simulink model "PMSM_5_foc_smo5k_2019b"  (R2016a)
settings: Solver=ode45  StartTime=0.0  StopTime=0.8  FixedStep=1e-6  RelTol=1e-2
undefined symbols (not defined in the file or in its folder): Ls, Rs, udc
libraries: powerlib x7, simulink x4, powerlib_meascontrol x4
settings Model: Creator=Administrator  LastModifiedBy=Administrator

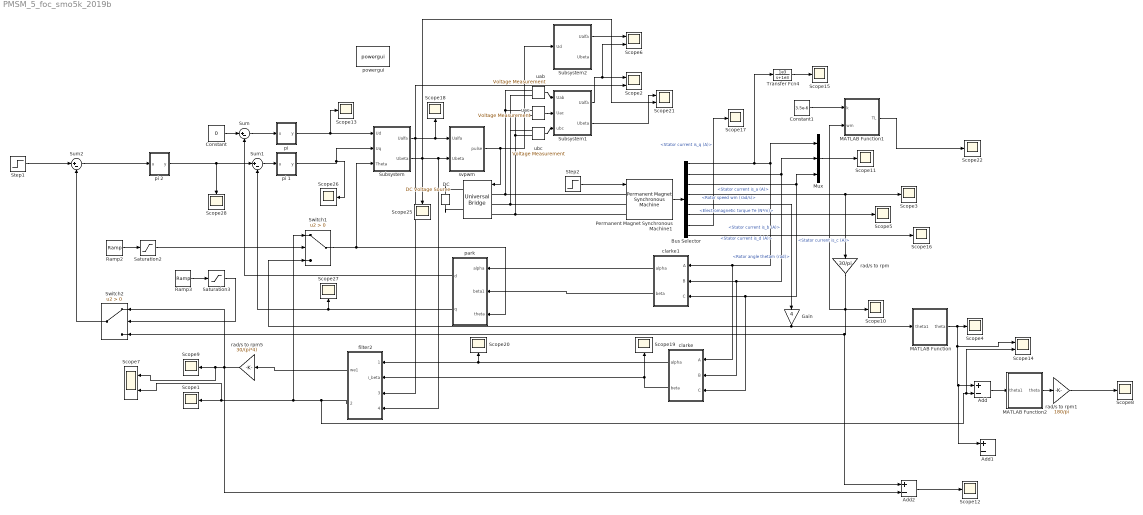
== system PMSM_5_foc_smo5k_2019b ==
  "   " : powerlib/Power Electronics/Universal Bridge  Arms=3  SnubberResistance=1e5  SnubberCapacitance=inf  Device=IGBT / Diodes  Ron=1e-3  Lon=0  ForwardVoltages="[  0  0  ]"  ForwardVoltage=0  GTOparameters=[ 10e-6 , 20e-6 ]  IGBTparameters=[ 1e-6 , 2e-6 ]  Measurements=All voltages and currents  Measurements_2=None  converterType=Rectifier
  " rad/s to rpm" : Gain  Gain=30/pi
  " rad/s to rpm1" : Gain  Gain=180/pi
  " rad/s to rpm5" : Gain  Gain=30/(pi*4)
  Add : Sum  Inputs=+-
  Add1 : Sum  Inputs=+-
  Add2 : Sum  Inputs=+-
  Bus Selector : BusSelector  OutputSignals=Stator current is_a (A),Stator current is_b (A),Stator current is_c (A),Rotor speed wm (rad/s),Rotor angle thetam (rad),Electromagnetic torque Te (N*m),Stator current is_q (A),Stator current is_d (A)
  Constant : Constant  Value=0
  Constant1 : Constant  Value=3.5e-6
  "DC " : powerlib/Electrical Sources/DC Voltage Source  Amplitude=280  Measurements=None
  Gain : Gain  Gain=4
  MATLAB Function : MATLAB Function  TreatAsAtomicUnit=on
  MATLAB Function1 : MATLAB Function  TreatAsAtomicUnit=on
  MATLAB Function2 : MATLAB Function  TreatAsAtomicUnit=on
  Mux : Mux  Inputs=3
  Permanent Magnet Synchronous Machine1 : powerlib/Machines/Permanent Magnet Synchronous Machine  NbPhases=3  FluxDistribution=Sinusoidal  RotorType=Salient-pole  MechanicalLoad=Torque Tm  PresetModel=No  ShowDetailedParameters=on  MeasurementBus=off  Resistance=0.1  Inductance=8.5e-3  dqInductances=[0.8e-3,0.8e-3]  La=1.6e-3  MachineConstant=Flux linkage established by magnets (V.s)  Flux=0.11  VoltageCst=79.8072  TorqueCst=0.66  Flat=120  Mechanical=[0.00223 0 4 0]  PolePairs=4  InitialConditions=[0,0, 0,0]  InitialConditions5ph=[0 0 0 0 0 0]  TsPowergui=0  TsBlock=-1  RefAngle=Aligned with phase A axis (original Park)
  Ramp2 : simulink/Sources/Ramp  slope=1  start=0  X0=-2
  Ramp3 : simulink/Sources/Ramp  slope=1  start=0  X0=-2
  Saturation2 : Saturate  UpperLimit=1  LowerLimit=0
  Saturation3 : Saturate  UpperLimit=1  LowerLimit=0
  Scope{1,3..5,8..13,15..20,22,25..28} (21 alike) : Scope
  Scope{2,6..7,14,21} (5 alike) : Scope  NumInputPorts=2
  Step1 : Step  Time=0.5  Before=400  After=400  SampleTime=0
  Step2 : Step  Time=0.3  Before=10  After=10  SampleTime=0
  Subsystem : Subsystem
  Subsystem1 : Subsystem
  Subsystem2 : Subsystem  InitFcn=udc=283
  Sum : Sum  Inputs=|+-
  Sum1 : Sum  Inputs=|+-
  Sum2 : Sum  Inputs=|+-
  Switch1 : Switch  Criteria=u2 > Threshold
  Switch2 : Switch  Criteria=u2 > Threshold
  Transfer Fcn4 : TransferFcn  Numerator=[1e3]  Denominator=[1 1e3]
  clarke : Subsystem
  clarke1 : Subsystem
  filter2 : Subsystem  InitFcn=|
      | Ls=0.8e-3
      | Rs=0.1
  park : Subsystem
  "pi " : Subsystem  mask{P=0.72, I=90, UpperSaturationLimit=280, LowerSaturationLimit=-280, SampleTime=-1}
  pi 1 : Subsystem  mask{P=0.72, I=90, UpperSaturationLimit=280, LowerSaturationLimit=-280, SampleTime=-1}
  pi 2 : Subsystem  mask{P=0.1061, I=10.6148, UpperSaturationLimit=30, LowerSaturationLimit=-30, SampleTime=-1}
  powergui : powerlib/powergui  Priority=1  SimulationMode=Continuous  SolverType=Backward Euler  SampleTime=1e-6  frequency=60  SPID=off  DisableSnubberDevices=off  DisableRonSwitches=off  DisableVfSwitches=off  SwTol=0  DisplayEquations=off  Interpol=off  ExternalGateDelay=off  methode=off  Ts=0  FunctionMessages=off  echomessages=off  HookPort=off  EnableUseOfTLC=off  x0status=blocks  frequencyindice=0  Pbase=100e6  ErrMax=1e-4  Iterations=50  UnitsV=kV  UnitsW=MW  buscounter=0  RestoreLinks=warning  ResistiveCurrentMeasurement=off  Frange=[0:2:500]  Ylog=off  Xlog=on  ShowGrid=off  save=off  variable=ZData  structure=smo5k_ia  ZoomFFT=off  StartTime=0.5  cycles=1  DisplayStyle=1  fundamental=200/3  FreqAxis=on  MaxFrequency=6000  frequencyindicesteady=1  RmsSteady=1  display=off
  svpwm : Subsystem  mask{T=1/2000, Udc=280, T_deadtime=0}
      mask prompts: T "T(s)"; Udc "Udc(V)"; T_deadtime "T_deadtime(us)"
  uab : powerlib/Measurements/Voltage Measurement  PhasorSimulation=off  OutputType=Complex  PSBequivalent=0
  uac : powerlib/Measurements/Voltage Measurement  PhasorSimulation=off  OutputType=Complex  PSBequivalent=0
  ubc : powerlib/Measurements/Voltage Measurement  PhasorSimulation=off  OutputType=Complex  PSBequivalent=0
  wires:
  svpwm/1(pulse) -> "   "/1, Subsystem2/1(Ud)
  Bus Selector/1 -> clarke/1(A), clarke1/1(A), Mux/1, Transfer Fcn4/1  "<Stator current is_a (A)>"
  Bus Selector/2 -> clarke/2(B), clarke1/2(B), Mux/2  "<Stator current is_b (A)>"
  Bus Selector/3 -> clarke/3(C), clarke1/3(C), Mux/3  "<Stator current is_c (A)>"
  Bus Selector/4 -> " rad/s to rpm"/1, Scope3/1  "<Rotor speed wm (rad/s)>"
  Bus Selector/5 -> Gain/1  "<Rotor angle thetam (rad)>"
  Bus Selector/6 -> Scope5/1  "<Electromagnetic torque Te (N*m)>"
  clarke/2(beta) -> Scope19/1, filter2/2(i_beta)
  Sum/1 -> "pi "/1(u)
  "pi "/1(y) -> Scope13/1, Subsystem/1(Ud)
  park/1(d) -> Sum/2
  Sum1/1 -> pi 1/1(u)
  Mux/1 -> Scope11/1
  Permanent Magnet Synchronous Machine1/1 -> Bus Selector/1
  Bus Selector/7 -> Scope17/1  "<Stator current is_q (A)>"
  Bus Selector/8 -> Scope16/1  "<Stator current is_d (A)>"
  Constant/1 -> Sum/1
  park/2(q) -> Sum1/2, Scope27/1
  pi 1/1(y) -> Scope26/1, Subsystem/2(Uq)
  pi 2/1(y) -> Sum1/1, Scope28/1
  filter2/1(we1) -> " rad/s to rpm5"/1
  Gain/1 -> MATLAB Function/1(theta1), Switch1/3
  " rad/s to rpm5"/1 -> Add2/2, Switch2/1, Scope7/1, Scope9/1
  filter2/2(theta*2) -> Scope14/2, Add/2, Switch1/1, Scope7/2, Scope1/1
  " rad/s to rpm"/1 -> MATLAB Function1/2(wm), Add2/1, Switch2/3, Scope10/1
  Step1/1 -> Sum2/1
  Switch2/1 -> Sum2/2
  Switch1/1 -> park/3(theta), Subsystem/3(Theta)
  Ramp2/1 -> Saturation2/1
  Saturation2/1 -> Switch1/2
  Ramp3/1 -> Saturation3/1
  Saturation3/1 -> Switch2/2
  clarke/1(alpha) -> Scope20/1, filter2/1(i_alpha)
  Transfer Fcn4/1 -> Scope15/1
  clarke1/1(alpha) -> park/1(alpha)
  clarke1/2(beta) -> park/2(beta1)
  uac/1 -> Subsystem1/2(Uac)
  uab/1 -> Subsystem1/1(Uab)
  ubc/1 -> Subsystem1/3(ubc)
  Subsystem1/1(Ualfa) -> Scope6/2, Scope2/1
  Subsystem1/2(Ubeta) -> Scope21/1
  Sum2/1 -> pi 2/1(u)
  Subsystem/1(Ualfa) -> svpwm/1(Ualfa), Scope18/1, filter2/3(u_alpha), Scope2/2
  Subsystem/2(Ubeta) -> Scope21/2, filter2/4(u_beta), svpwm/2(Ubeta), Scope25/1
  Step2/1 -> Permanent Magnet Synchronous Machine1/1
  Constant1/1 -> MATLAB Function1/1(k)
  MATLAB Function1/1(TL) -> Scope22/1
  Subsystem2/1(Ualfa) -> Scope6/1
  Add/1 -> MATLAB Function2/1(theta1)
  MATLAB Function/1(theta) -> Scope14/1, Add1/1, Add/1, Scope4/1
  Add2/1 -> Scope12/1
  MATLAB Function2/1(theta) -> " rad/s to rpm1"/1
  " rad/s to rpm1"/1 -> Scope8/1
  connections:
  "DC "/RConn1 -- "   "/RConn1
  Permanent Magnet Synchronous Machine1/LConn1 -- uab/LConn1 -- uac/LConn1 -- "   "/LConn1
  "DC "/LConn1 -- "   "/RConn2
  Permanent Magnet Synchronous Machine1/LConn3 -- ubc/LConn2 -- uac/LConn2 -- "   "/LConn3
  Permanent Magnet Synchronous Machine1/LConn2 -- ubc/LConn1 -- uab/LConn2 -- "   "/LConn2

== system PMSM_5_foc_smo5k_2019b/Subsystem ==
  Ud : Inport
  Uq : Inport  Port=2
  Theta : Inport  Port=3
  Fcn : Fcn  Expr=u(1)*cos(u(3))-u(2)*sin(u(3))
  Fcn1 : Fcn  Expr=u(1)*sin(u(3))+u(2)*cos(u(3))
  Mux : Mux  Inputs=3
  Mux1 : Mux  Inputs=3
  Ualfa : Outport
  Ubeta : Outport  Port=2
  wires:
  Ud/1 -> Mux1/1, Mux/1
  Uq/1 -> Mux1/2, Mux/2
  Theta/1 -> Mux1/3, Mux/3
  Mux/1 -> Fcn/1
  Mux1/1 -> Fcn1/1
  Fcn/1 -> Ualfa/1
  Fcn1/1 -> Ubeta/1

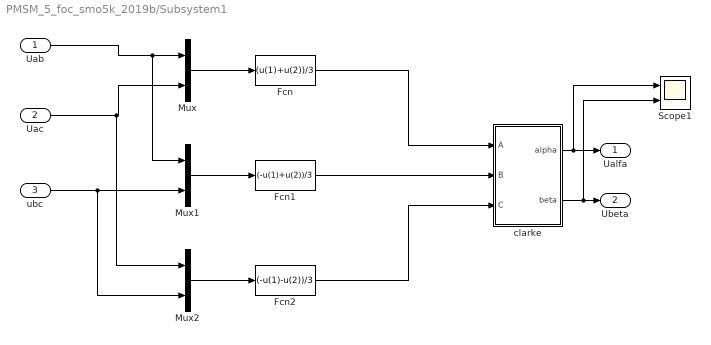
== system PMSM_5_foc_smo5k_2019b/Subsystem1 ==
  Uab : Inport
  Uac : Inport  Port=2
  ubc : Inport  Port=3
  Fcn : Fcn  Expr=(u(1)+u(2))/3
  Fcn1 : Fcn  Expr=(-u(1)+u(2))/3
  Fcn2 : Fcn  Expr=(-u(1)-u(2))/3
  Mux : Mux  Inputs=2
  Mux1 : Mux  Inputs=2
  Mux2 : Mux  Inputs=2
  Scope1 : Scope  NumInputPorts=2
  clarke : Subsystem
  Ualfa : Outport
  Ubeta : Outport  Port=2
  wires:
  Mux/1 -> Fcn/1
  Fcn/1 -> clarke/1(A)
  Mux1/1 -> Fcn1/1
  Fcn1/1 -> clarke/2(B)
  Uab/1 -> Mux1/1, Mux/1
  Mux2/1 -> Fcn2/1
  Fcn2/1 -> clarke/3(C)
  Uac/1 -> Mux2/1, Mux/2
  ubc/1 -> Mux2/2, Mux1/2
  clarke/2(beta) -> Scope1/2, Ubeta/1
  clarke/1(alpha) -> Scope1/1, Ualfa/1

== system PMSM_5_foc_smo5k_2019b/Subsystem2 ==
  Ud : Inport
  Demux : Demux  Outputs=6
  Fcn : Fcn  Expr=u(1)-u(2)-u(3)+u(4)
  Fcn1 : Fcn  Expr=u(1)-u(2)-u(5)+u(6)
  Fcn2 : Fcn  Expr=u(3)-u(4)-u(5)+u(6)
  Gain : Gain  Gain=udc/2
  Gain1 : Gain  Gain=udc/2
  Gain2 : Gain  Gain=udc/2
  Mux : Mux  Inputs=6
  Subsystem1 : Subsystem
  Ualfa : Outport
  Ubeta : Outport  Port=2
  wires:
  Ud/1 -> Demux/1
  Demux/1 -> Mux/1
  Demux/2 -> Mux/2
  Demux/3 -> Mux/3
  Demux/4 -> Mux/4
  Demux/5 -> Mux/5
  Demux/6 -> Mux/6
  Mux/1 -> Fcn2/1, Fcn1/1, Fcn/1
  Fcn/1 -> Gain/1
  Fcn1/1 -> Gain1/1
  Fcn2/1 -> Gain2/1
  Subsystem1/1(Ualfa) -> Ualfa/1
  Subsystem1/2(Ubeta) -> Ubeta/1
  Gain/1 -> Subsystem1/1(Uab)
  Gain2/1 -> Subsystem1/3(ubc)
  Gain1/1 -> Subsystem1/2(Uac)

== system PMSM_5_foc_smo5k_2019b/clarke ==
  A : Inport
  B : Inport  Port=2
  C : Inport  Port=3
  Fcn : Fcn  Expr=2/3*(u(1)-(1/2)*u(2)-(1/2)*u(3))
  Fcn1 : Fcn  Expr=2/3*(0*u(1)+(sqrt(3)/2)*u(2)-(sqrt(3)/2)*u(3))
  Mux : Mux  Inputs=3
  Mux1 : Mux  Inputs=3
  alpha : Outport
  beta : Outport  Port=2
  wires:
  Fcn/1 -> alpha/1
  Fcn1/1 -> beta/1
  A/1 -> Mux1/1, Mux/1
  B/1 -> Mux/2, Mux1/2
  C/1 -> Mux/3, Mux1/3
  Mux/1 -> Fcn/1
  Mux1/1 -> Fcn1/1

== system PMSM_5_foc_smo5k_2019b/clarke1 ==
  A : Inport
  B : Inport  Port=2
  C : Inport  Port=3
  Fcn : Fcn  Expr=2/3*(u(1)-(1/2)*u(2)-(1/2)*u(3))
  Fcn1 : Fcn  Expr=2/3*(0*u(1)+(sqrt(3)/2)*u(2)-(sqrt(3)/2)*u(3))
  Mux : Mux  Inputs=3
  Mux1 : Mux  Inputs=3
  alpha : Outport
  beta : Outport  Port=2
  wires:
  Fcn/1 -> alpha/1
  Fcn1/1 -> beta/1
  A/1 -> Mux1/1, Mux/1
  B/1 -> Mux/2, Mux1/2
  C/1 -> Mux/3, Mux1/3
  Mux/1 -> Fcn/1
  Mux1/1 -> Fcn1/1

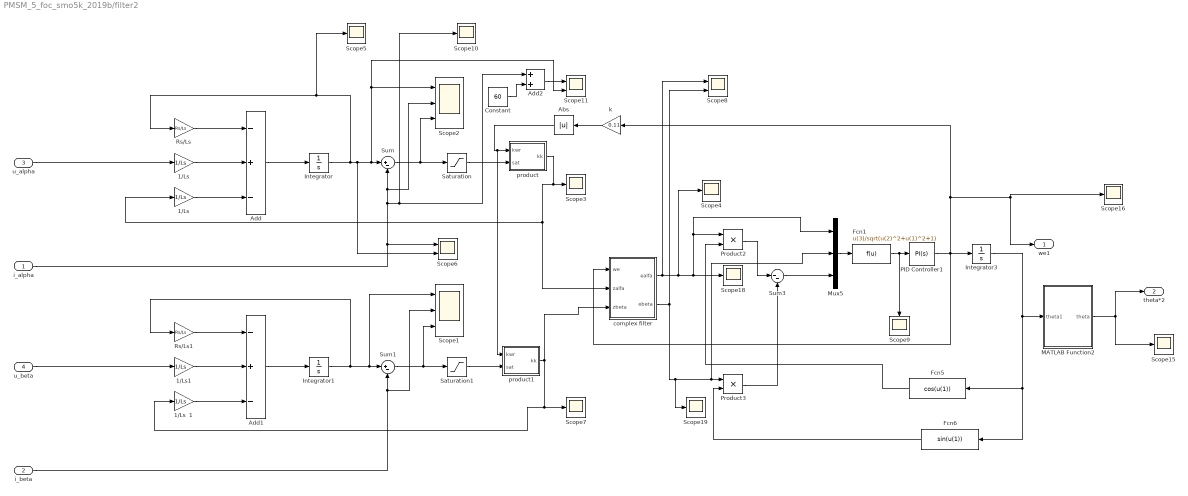
== system PMSM_5_foc_smo5k_2019b/filter2 ==
  i_alpha : Inport
  i_beta : Inport  Port=2
  u_alpha : Inport  Port=3
  u_beta : Inport  Port=4
  " product" : MATLAB Function  TreatAsAtomicUnit=on
  " product1" : MATLAB Function  TreatAsAtomicUnit=on
  1/Ls : Gain  Gain=1/Ls
  "1/Ls  " : Gain  Gain=1/Ls
  1/Ls  1 : Gain  Gain=1/Ls
  1/Ls1 : Gain  Gain=1/Ls
  Abs : Abs
  Add : Sum  Inputs=-+-
  Add1 : Sum  Inputs=-+-
  Add2 : Sum
  Constant : Constant  Value=60
  Fcn1 : Fcn  Expr=u(3)/sqrt(u(2)^2+u(1)^2+1)
  Fcn5 : Fcn  Expr=cos(u(1))
  Fcn6 : Fcn  Expr=sin(u(1))
  Integrator : Integrator
  Integrator1 : Integrator
  Integrator3 : Integrator
  MATLAB Function2 : MATLAB Function  TreatAsAtomicUnit=on
  Mux5 : Mux  Inputs=3
  PID Controller1 : simulink/Continuous/PID Controller  Controller=PI  TimeDomain=Continuous-time  SampleTime=-1  IntegratorMethod=Forward Euler  FilterMethod=Forward Euler  Form=Parallel  UseFilter=on  ControllerParametersSource=internal  P=200  I=10000  D=0  N=100  InitialConditionSource=internal  InitialConditionForIntegrator=0  InitialConditionForFilter=0  ExternalReset=none  LimitOutput=off  UpperSaturationLimit=1000  LowerSaturationLimit=-1000  LinearizeAsGain=on  AntiWindupMode=none  Kb=1  TrackingMode=off  Kt=1  PParamMin=[]  PParamMax=[]  IParamMin=[]  IParamMax=[]  DParamMin=[]  DParamMax=[]  NParamMin=[]  NParamMax=[]  KbParamMin=[]  KbParamMax=[]  KtParamMin=[]  KtParamMax=[]  POutMin=[]  POutMax=[]  IOutMin=[]  IOutMax=[]  DOutMin=[]  DOutMax=[]  NOutMin=[]  NOutMax=[]  KbOutMin=[]  KbOutMax=[]  KtOutMin=[]  KtOutMax=[]  IntegratorOutMin=[]  IntegratorOutMax=[]  FilterOutMin=[]  FilterOutMax=[]  SumOutMin=[]  SumOutMax=[]  SumI1OutMin=[]  SumI1OutMax=[]  SumI2OutMin=[]  SumI2OutMax=[]  SumI3OutMin=[]  SumI3OutMax=[]  SumDOutMin=[]  SumDOutMax=[]  SaturationOutMin=[]  SaturationOutMax=[]  IntegratorContinuousStateAttributes=''  IntegratorStateMustResolveToSignalObject=off  IntegratorRTWStateStorageClass=Auto  FilterContinuousStateAttributes=''  FilterStateMustResolveToSignalObject=off  FilterRTWStateStorageClass=Auto  DifferentiatorICPrevScaledInput=0  DifferentiatorOutMin=[]  DifferentiatorOutMax=[]
  Product2 : Product
  Product3 : Product
  Rs/Ls : Gain  Gain=Rs/Ls
  Rs/Ls1 : Gain  Gain=Rs/Ls
  Saturation : Saturate  UpperLimit=1  LowerLimit=-1
  Saturation1 : Saturate  UpperLimit=1  LowerLimit=-1
  Scope1 : Scope  NumInputPorts=3
  Scope{3..5,7,9..10,15..16,18..19} (10 alike) : Scope
  Scope11 : Scope  NumInputPorts=2
  Scope2 : Scope  NumInputPorts=3
  Scope6 : Scope  NumInputPorts=2
  Scope8 : Scope  NumInputPorts=2
  Sum : Sum  Inputs=|+-
  Sum1 : Sum  Inputs=|+-
  Sum3 : Sum  Inputs=|--
  complex filter : Subsystem  mask{k_ccf=2}
  k : Gain  Gain=0.11
  we1 : Outport
  theta*2 : Outport  Port=2
  wires:
  Rs/Ls/1 -> Add/1
  1/Ls/1 -> Add/2
  Add/1 -> Integrator/1
  Integrator/1 -> Scope5/1, Rs/Ls/1, Scope6/2, Scope11/2, Scope2/1, Sum/1
  "1/Ls  "/1 -> Add/3
  Rs/Ls1/1 -> Add1/1
  1/Ls1/1 -> Add1/2
  Add1/1 -> Integrator1/1
  1/Ls  1/1 -> Add1/3
  complex filter/2(ebeta) -> Scope19/1, Product3/1, Mux5/2, Scope8/2
  Product2/1 -> Sum3/1
  Product3/1 -> Sum3/2
  Fcn6/1 -> Product3/2
  Fcn5/1 -> Product2/2
  Integrator3/1 -> MATLAB Function2/1(theta1), Fcn6/1, Fcn5/1
  Mux5/1 -> Fcn1/1
  Sum3/1 -> Mux5/3
  Fcn1/1 -> Scope9/1, PID Controller1/1
  PID Controller1/1 -> k/1, we1/1, Scope16/1, complex filter/1(we), Integrator3/1
  MATLAB Function2/1(theta) -> theta*2/1, Scope15/1
  Saturation1/1 -> " product1"/2(sat)
  Integrator1/1 -> Rs/Ls1/1, Scope1/1, Sum1/1
  Saturation/1 -> " product"/2(sat)
  " product"/1(kk) -> complex filter/2(zalfa), "1/Ls  "/1, Scope3/1
  " product1"/1(kk) -> 1/Ls  1/1, Scope7/1, complex filter/3(zbeta)
  Sum/1 -> Scope2/3, Saturation/1
  Sum1/1 -> Scope1/3, Saturation1/1
  u_alpha/1 -> 1/Ls/1
  i_alpha/1 -> Add2/1, Scope10/1, Scope2/2, Sum/2, Scope6/1
  u_beta/1 -> 1/Ls1/1
  i_beta/1 -> Scope1/2, Sum1/2
  k/1 -> Abs/1
  complex filter/1(ealfa) -> Scope8/1, Scope4/1, Mux5/1, Product2/1, Scope18/1
  Constant/1 -> Add2/2
  Add2/1 -> Scope11/1
  Abs/1 -> " product1"/1(kwr), " product"/1(kwr)

== system PMSM_5_foc_smo5k_2019b/park ==
  alpha : Inport
  beta1 : Inport  Port=2
  theta : Inport  Port=3
  Fcn : Fcn  Expr=cos(u(3))*u(1)+sin(u(3))*u(2)
  Fcn1 : Fcn  Expr=-sin(u(3))*u(1)+cos(u(3))*u(2)
  Mux : Mux  Inputs=3
  Mux1 : Mux  Inputs=3
  d : Outport
  q : Outport  Port=2
  wires:
  Mux/1 -> Fcn/1
  Mux1/1 -> Fcn1/1
  Fcn/1 -> d/1
  Fcn1/1 -> q/1
  alpha/1 -> Mux1/1, Mux/1
  beta1/1 -> Mux/2, Mux1/2
  theta/1 -> Mux/3, Mux1/3

== system PMSM_5_foc_smo5k_2019b/pi  ==
  u : Inport
  Constant : Constant  Commented=on
  I : Gain  Gain=I
  Integrator1 : Integrator
  Logical Operator : Logic  Commented=on  AllPortsSameDT=off  OutDataTypeStr=boolean
  MATLAB Function1 : MATLAB Function  TreatAsAtomicUnit=on
  MATLAB Function2 : MATLAB Function  TreatAsAtomicUnit=on
  P : Gain  Gain=P
  Saturate : Saturate  UpperLimit=UpperSaturationLimit  LowerLimit=LowerSaturationLimit
  Sum3 : Sum  Inputs=++|  SampleTime=SampleTime
  Switch : Switch  Commented=on  Criteria=u2 > Threshold
  y : Outport  SampleTime=SampleTime  InitialOutput=0
  wires:
  u/1 -> P/1, MATLAB Function2/4(error)
  I/1 -> Integrator1/1
  Integrator1/1 -> Sum3/2
  P/1 -> Sum3/1
  Saturate/1 -> MATLAB Function1/2(y2), y/1
  Sum3/1 -> MATLAB Function1/1(y1), Saturate/1
  Constant/1 -> Logical Operator/2
  MATLAB Function1/1(postive_flag) -> MATLAB Function2/1(postive_flag)
  MATLAB Function1/2(negative_flag) -> MATLAB Function2/2(negative_flag)
  MATLAB Function1/3(flag) -> MATLAB Function2/3(flag)
  MATLAB Function2/1(out) -> I/1

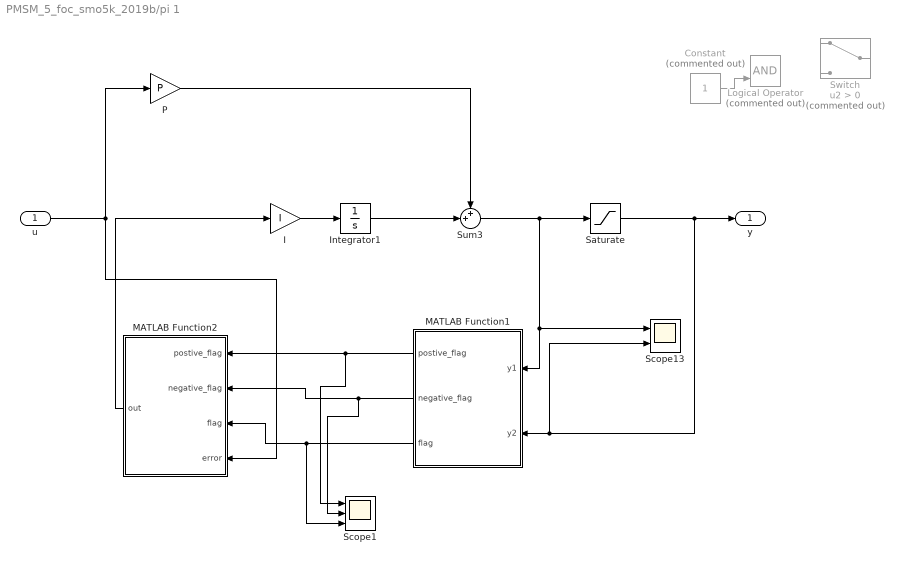
== system PMSM_5_foc_smo5k_2019b/pi 1 ==
  u : Inport
  Constant : Constant  Commented=on
  I : Gain  Gain=I
  Integrator1 : Integrator
  Logical Operator : Logic  Commented=on  AllPortsSameDT=off  OutDataTypeStr=boolean
  MATLAB Function1 : MATLAB Function  TreatAsAtomicUnit=on
  MATLAB Function2 : MATLAB Function  TreatAsAtomicUnit=on
  P : Gain  Gain=P
  Saturate : Saturate  UpperLimit=UpperSaturationLimit  LowerLimit=LowerSaturationLimit
  Scope1 : Scope  NumInputPorts=3
  Scope13 : Scope  NumInputPorts=2
  Sum3 : Sum  Inputs=++|  SampleTime=SampleTime
  Switch : Switch  Commented=on  Criteria=u2 > Threshold
  y : Outport  SampleTime=SampleTime  InitialOutput=0
  wires:
  u/1 -> P/1, MATLAB Function2/4(error)
  I/1 -> Integrator1/1
  Integrator1/1 -> Sum3/2
  P/1 -> Sum3/1
  Saturate/1 -> Scope13/2, MATLAB Function1/2(y2), y/1
  Sum3/1 -> Scope13/1, MATLAB Function1/1(y1), Saturate/1
  Constant/1 -> Logical Operator/2
  MATLAB Function1/1(postive_flag) -> Scope1/1, MATLAB Function2/1(postive_flag)
  MATLAB Function1/2(negative_flag) -> Scope1/2, MATLAB Function2/2(negative_flag)
  MATLAB Function1/3(flag) -> Scope1/3, MATLAB Function2/3(flag)
  MATLAB Function2/1(out) -> I/1

== system PMSM_5_foc_smo5k_2019b/pi 2 ==
  u : Inport
  Constant : Constant  Commented=on
  I : Gain  Gain=I
  Integrator1 : Integrator
  Logical Operator : Logic  Commented=on  AllPortsSameDT=off  OutDataTypeStr=boolean
  MATLAB Function1 : MATLAB Function  TreatAsAtomicUnit=on
  MATLAB Function2 : MATLAB Function  TreatAsAtomicUnit=on
  P : Gain  Gain=P
  Saturate : Saturate  UpperLimit=UpperSaturationLimit  LowerLimit=LowerSaturationLimit  ZeroCross=off
  Sum3 : Sum  Inputs=++|  SampleTime=SampleTime
  Switch : Switch  Commented=on  Criteria=u2 > Threshold
  y : Outport  SampleTime=SampleTime  InitialOutput=0
  wires:
  I/1 -> Integrator1/1
  Integrator1/1 -> Sum3/2
  P/1 -> Sum3/1
  Saturate/1 -> MATLAB Function1/2(y2), y/1
  Sum3/1 -> MATLAB Function1/1(y1), Saturate/1
  Constant/1 -> Logical Operator/2
  MATLAB Function1/1(postive_flag) -> MATLAB Function2/1(postive_flag)
  MATLAB Function1/2(negative_flag) -> MATLAB Function2/2(negative_flag)
  MATLAB Function1/3(flag) -> MATLAB Function2/3(flag)
  u/1 -> P/1, MATLAB Function2/4(error)
  MATLAB Function2/1(out) -> I/1

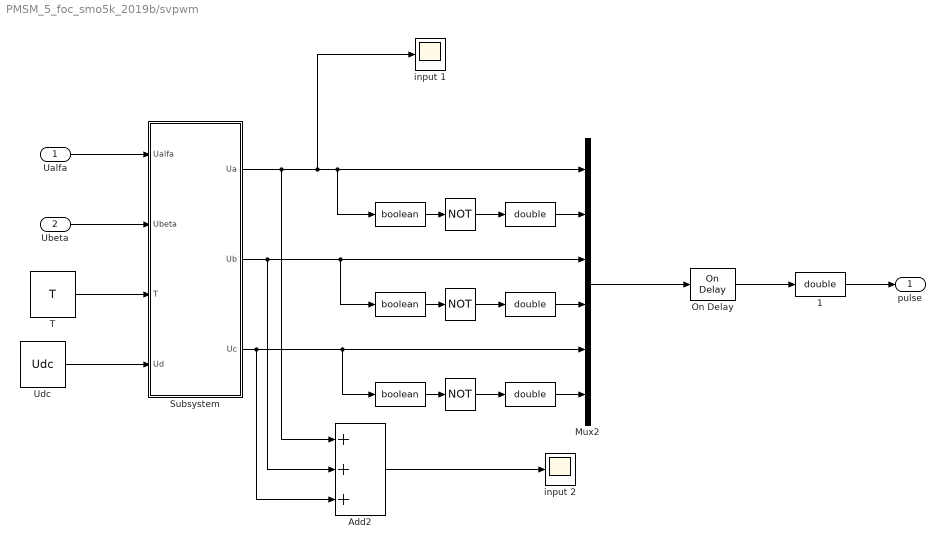
== system PMSM_5_foc_smo5k_2019b/svpwm ==
  Ualfa : Inport
  Ubeta : Inport  Port=2
  " " : DataTypeConversion  OutDataTypeStr=boolean
  "   " : DataTypeConversion  OutDataTypeStr=boolean
  "    " : DataTypeConversion  OutDataTypeStr=boolean
  "      " : DataTypeConversion  OutDataTypeStr=double
  " " : Logic  Operator=NOT  Inputs=1  AllPortsSameDT=off  OutDataTypeStr=boolean
  "        " : DataTypeConversion  OutDataTypeStr=double
  "           " : Logic  Operator=NOT  Inputs=1  AllPortsSameDT=off  OutDataTypeStr=boolean
  "            " : Logic  Operator=NOT  Inputs=1  AllPortsSameDT=off  OutDataTypeStr=boolean
  "                          " : DataTypeConversion  OutDataTypeStr=double
  "                          1" : DataTypeConversion  OutDataTypeStr=double
  Add2 : Sum  Inputs=+++
  Mux2 : Mux  Inputs=6
  On Delay : powerlib_meascontrol/Logic/On Delay  DelayType=On delay  delay=T_deadtime*1e-6  ic=0  Ts=0
  Subsystem : Subsystem
  T : Constant  Value=T
  Udc : Constant  Value=Udc
  input 1 : Scope
  input 2 : Scope
  pulse : Outport
  wires:
  Mux2/1 -> On Delay/1
  Add2/1 -> input 2/1
  T/1 -> Subsystem/3(T)
  Udc/1 -> Subsystem/4(Ud)
  Ualfa/1 -> Subsystem/1(Ualfa)
  Ubeta/1 -> Subsystem/2(Ubeta)
  Subsystem/2(Ub) -> Add2/2, " "/1, Mux2/3
  Subsystem/3(Uc) -> Add2/3, "    "/1, Mux2/5
  "   "/1 -> "           "/1
  "           "/1 -> "                          "/1
  "                          "/1 -> Mux2/2
  " "/1 -> "            "/1
  "            "/1 -> "        "/1
  "        "/1 -> Mux2/4
  "    "/1 -> " "/1
  " "/1 -> "      "/1
  "      "/1 -> Mux2/6
  Subsystem/1(Ua) -> Add2/1, input 1/1, "   "/1, Mux2/1
  On Delay/1 -> "                          1"/1
  "                          1"/1 -> pulse/1

== system PMSM_5_foc_smo5k_2019b/Subsystem1/clarke ==
  A : Inport
  B : Inport  Port=2
  C : Inport  Port=3
  Fcn : Fcn  Expr=2/3*(u(1)-(1/2)*u(2)-(1/2)*u(3))
  Fcn1 : Fcn  Expr=2/3*(0*u(1)+(sqrt(3)/2)*u(2)-(sqrt(3)/2)*u(3))
  Mux : Mux  Inputs=3
  Mux1 : Mux  Inputs=3
  alpha : Outport
  beta : Outport  Port=2
  wires:
  Fcn/1 -> alpha/1
  Fcn1/1 -> beta/1
  A/1 -> Mux1/1, Mux/1
  B/1 -> Mux/2, Mux1/2
  C/1 -> Mux/3, Mux1/3
  Mux/1 -> Fcn/1
  Mux1/1 -> Fcn1/1

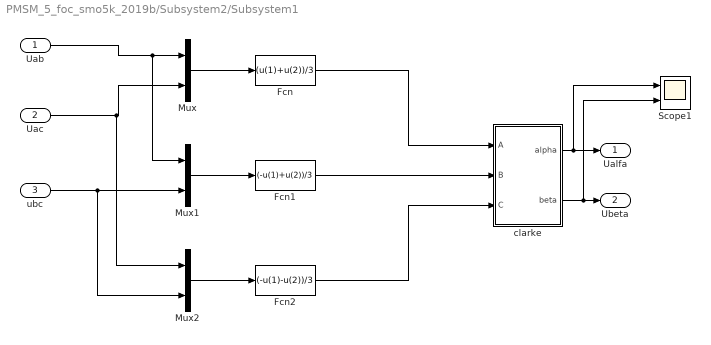
== system PMSM_5_foc_smo5k_2019b/Subsystem2/Subsystem1 ==
  Uab : Inport
  Uac : Inport  Port=2
  ubc : Inport  Port=3
  Fcn : Fcn  Expr=(u(1)+u(2))/3
  Fcn1 : Fcn  Expr=(-u(1)+u(2))/3
  Fcn2 : Fcn  Expr=(-u(1)-u(2))/3
  Mux : Mux  Inputs=2
  Mux1 : Mux  Inputs=2
  Mux2 : Mux  Inputs=2
  Scope1 : Scope  NumInputPorts=2
  clarke : Subsystem
  Ualfa : Outport
  Ubeta : Outport  Port=2
  wires:
  Mux/1 -> Fcn/1
  Fcn/1 -> clarke/1(A)
  Mux1/1 -> Fcn1/1
  Fcn1/1 -> clarke/2(B)
  Uab/1 -> Mux1/1, Mux/1
  Mux2/1 -> Fcn2/1
  Fcn2/1 -> clarke/3(C)
  Uac/1 -> Mux2/1, Mux/2
  ubc/1 -> Mux2/2, Mux1/2
  clarke/2(beta) -> Scope1/2, Ubeta/1
  clarke/1(alpha) -> Scope1/1, Ualfa/1

== system PMSM_5_foc_smo5k_2019b/filter2/complex filter ==
  we : Inport
  zalfa : Inport  Port=2
  zbeta : Inport  Port=3
  Constant : Constant  Value=k_ccf
  Integrator1 : Integrator
  Integrator3 : Integrator
  ccf : MATLAB Function  TreatAsAtomicUnit=on
  ealfa : Outport
  ebeta : Outport  Port=2
  wires:
  we/1 -> ccf/1(we_input)
  zalfa/1 -> ccf/2(ealfa)
  zbeta/1 -> ccf/3(ebeta)
  ccf/1(syalfa) -> Integrator3/1
  Integrator3/1 -> ccf/4(yalfa), ealfa/1
  ccf/2(sybeta) -> Integrator1/1
  Integrator1/1 -> ebeta/1, ccf/5(ybeta)
  Constant/1 -> ccf/6(k_ccf)

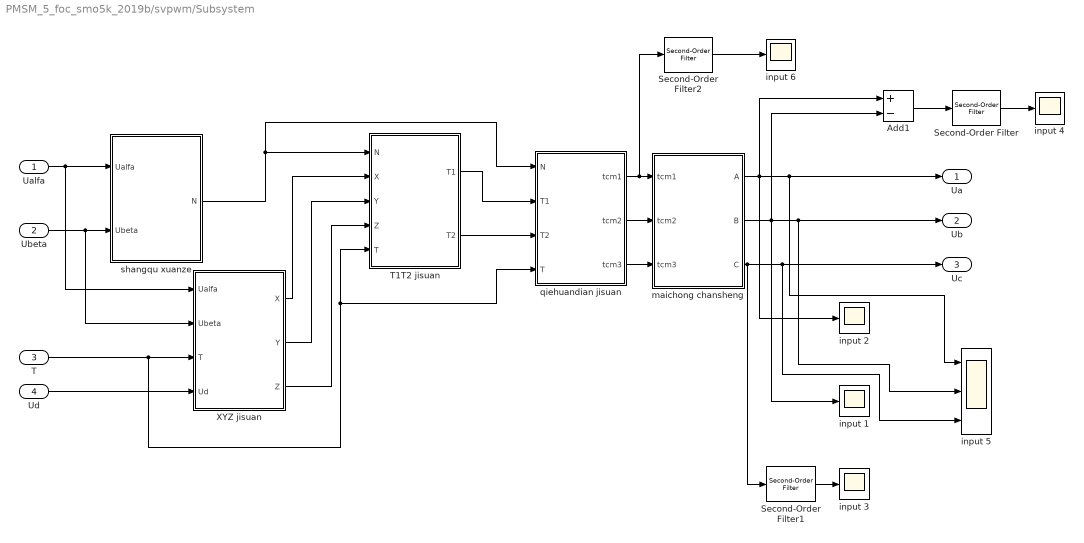
== system PMSM_5_foc_smo5k_2019b/svpwm/Subsystem ==
  Ualfa : Inport
  Ubeta : Inport  Port=2
  T : Inport  Port=3
  Ud : Inport  Port=4
  Add1 : Sum  Inputs=+-
  Second-Order Filter : powerlib_meascontrol/Filters/Second-Order Filter  FilterType=Lowpass  Fo=120  Zeta=0.707  Ts=0  Initialize=on  Vac_Init="[0,  0,  60]"  Vdc_Init=0  PlotResponse=off  FreqRange=[0, 500, 1]
  Second-Order Filter1 : powerlib_meascontrol/Filters/Second-Order Filter  FilterType=Lowpass  Fo=120  Zeta=0.707  Ts=0  Initialize=on  Vac_Init="[0,  0,  60]"  Vdc_Init=0  PlotResponse=off  FreqRange=[0, 500, 1]
  Second-Order Filter2 : powerlib_meascontrol/Filters/Second-Order Filter  FilterType=Lowpass  Fo=400  Zeta=0.707  Ts=0  Initialize=on  Vac_Init="[0,  0,  60]"  Vdc_Init=0  PlotResponse=off  FreqRange=[0, 500, 1]
  T1T2 jisuan : Subsystem
  XYZ jisuan : Subsystem
  input {1..4,6} (5 alike) : Scope
  input 5 : Scope  NumInputPorts=3
  maichong chansheng : Subsystem
  qiehuandian jisuan : Subsystem
  shangqu xuanze : Subsystem
  Ua : Outport
  Ub : Outport  Port=2
  Uc : Outport  Port=3
  wires:
  Ualfa/1 -> shangqu xuanze/1(Ualfa), XYZ jisuan/1(Ualfa)
  Ubeta/1 -> XYZ jisuan/2(Ubeta), shangqu xuanze/2(Ubeta)
  T/1 -> T1T2 jisuan/5(T), qiehuandian jisuan/4(T), XYZ jisuan/3(T)
  Ud/1 -> XYZ jisuan/4(Ud)
  shangqu xuanze/1(N) -> qiehuandian jisuan/1(N), T1T2 jisuan/1(N)
  XYZ jisuan/1(X) -> T1T2 jisuan/2(X)
  XYZ jisuan/2(Y) -> T1T2 jisuan/3(Y)
  XYZ jisuan/3(Z) -> T1T2 jisuan/4(Z)
  T1T2 jisuan/1(T1) -> qiehuandian jisuan/2(T1)
  T1T2 jisuan/2(T2) -> qiehuandian jisuan/3(T2)
  maichong chansheng/1(A) -> input 2/1, Ua/1, input 5/1, Add1/1
  qiehuandian jisuan/1(tcm1) -> Second-Order Filter2/1, maichong chansheng/1(tcm1)
  qiehuandian jisuan/2(tcm2) -> maichong chansheng/2(tcm2)
  qiehuandian jisuan/3(tcm3) -> maichong chansheng/3(tcm3)
  Add1/1 -> Second-Order Filter/1
  Second-Order Filter/1 -> input 4/1
  Second-Order Filter1/1 -> input 3/1
  maichong chansheng/3(C) -> Second-Order Filter1/1, Uc/1, input 5/3
  maichong chansheng/2(B) -> input 1/1, Ub/1, input 5/2, Add1/2
  Second-Order Filter2/1 -> input 6/1

== system PMSM_5_foc_smo5k_2019b/Subsystem2/Subsystem1/clarke ==
  A : Inport
  B : Inport  Port=2
  C : Inport  Port=3
  Fcn : Fcn  Expr=2/3*(u(1)-(1/2)*u(2)-(1/2)*u(3))
  Fcn1 : Fcn  Expr=2/3*(0*u(1)+(sqrt(3)/2)*u(2)-(sqrt(3)/2)*u(3))
  Mux : Mux  Inputs=3
  Mux1 : Mux  Inputs=3
  alpha : Outport
  beta : Outport  Port=2
  wires:
  Fcn/1 -> alpha/1
  Fcn1/1 -> beta/1
  A/1 -> Mux1/1, Mux/1
  B/1 -> Mux/2, Mux1/2
  C/1 -> Mux/3, Mux1/3
  Mux/1 -> Fcn/1
  Mux1/1 -> Fcn1/1

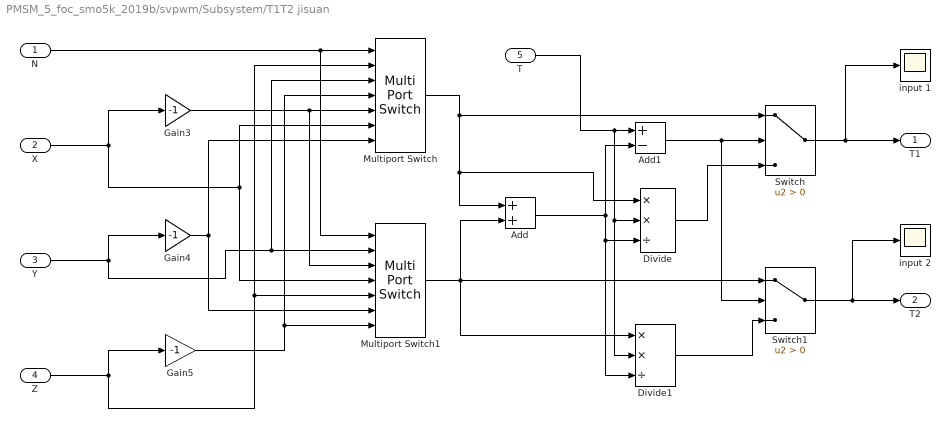
== system PMSM_5_foc_smo5k_2019b/svpwm/Subsystem/T1T2 jisuan ==
  N : Inport
  X : Inport  Port=2
  Y : Inport  Port=3
  Z : Inport  Port=4
  T : Inport  Port=5
  Add : Sum
  Add1 : Sum  Inputs=+-
  Divide : Product  Inputs=**/
  Divide1 : Product  Inputs=**/
  Gain3 : Gain  Gain=-1
  Gain4 : Gain  Gain=-1
  Gain5 : Gain  Gain=-1
  Multiport Switch : MultiPortSwitch  Inputs=6  DiagnosticForDefault=Warning
  Multiport Switch1 : MultiPortSwitch  Inputs=6  DiagnosticForDefault=Warning
  Switch : Switch  Criteria=u2 > Threshold
  Switch1 : Switch  Criteria=u2 > Threshold
  input 1 : Scope
  input 2 : Scope
  T1 : Outport
  T2 : Outport  Port=2
  wires:
  X/1 -> Gain3/1, Multiport Switch1/4, Multiport Switch/6
  Y/1 -> Multiport Switch1/2, Multiport Switch/3, Gain4/1
  N/1 -> Multiport Switch1/1, Multiport Switch/1
  Z/1 -> Gain5/1, Multiport Switch1/5, Multiport Switch/2
  Multiport Switch/1 -> Add/1, Divide/1, Switch/1
  Multiport Switch1/1 -> Divide1/1, Add/2, Switch1/1
  T/1 -> Add1/1, Divide/2, Divide1/2
  Add1/1 -> Switch1/2, Switch/2
  Add/1 -> Add1/2, Divide/3, Divide1/3
  Divide/1 -> Switch/3
  Divide1/1 -> Switch1/3
  Switch/1 -> input 1/1, T1/1
  Switch1/1 -> input 2/1, T2/1
  Gain3/1 -> Multiport Switch1/3, Multiport Switch/5
  Gain5/1 -> Multiport Switch1/7, Multiport Switch/4
  Gain4/1 -> Multiport Switch/7, Multiport Switch1/6

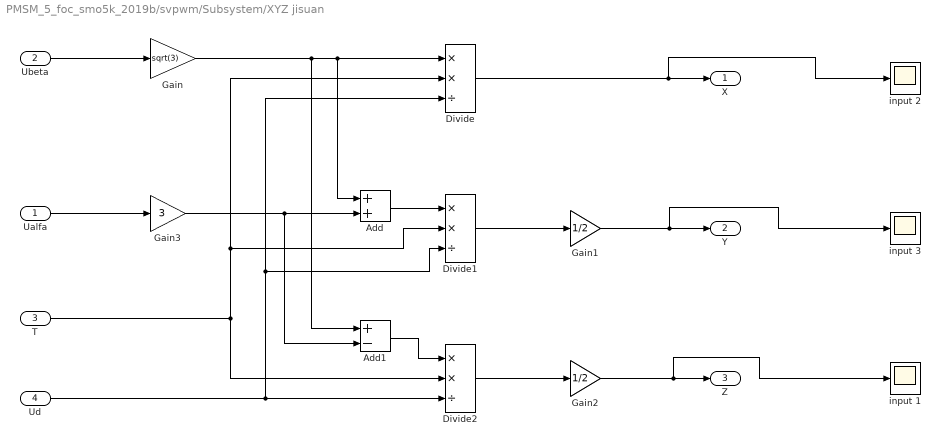
== system PMSM_5_foc_smo5k_2019b/svpwm/Subsystem/XYZ jisuan ==
  Ualfa : Inport
  Ubeta : Inport  Port=2
  T : Inport  Port=3
  Ud : Inport  Port=4
  Add : Sum
  Add1 : Sum  Inputs=+-
  Divide : Product  Inputs=**/
  Divide1 : Product  Inputs=**/
  Divide2 : Product  Inputs=**/
  Gain : Gain  Gain=sqrt(3)
  Gain1 : Gain  Gain=1/2
  Gain2 : Gain  Gain=1/2
  Gain3 : Gain  Gain=3
  input 1 : Scope
  input 2 : Scope
  input 3 : Scope
  X : Outport
  Y : Outport  Port=2
  Z : Outport  Port=3
  wires:
  Divide/1 -> input 2/1, X/1
  Ubeta/1 -> Gain/1
  Gain/1 -> Add1/1, Add/1, Divide/1
  T/1 -> Divide1/2, Divide/2, Divide2/2
  Ud/1 -> Divide2/3, Divide1/3, Divide/3
  Ualfa/1 -> Gain3/1
  Gain3/1 -> Add1/2, Add/2
  Add/1 -> Divide1/1
  Divide1/1 -> Gain1/1
  Gain1/1 -> input 3/1, Y/1
  Add1/1 -> Divide2/1
  Divide2/1 -> Gain2/1
  Gain2/1 -> input 1/1, Z/1

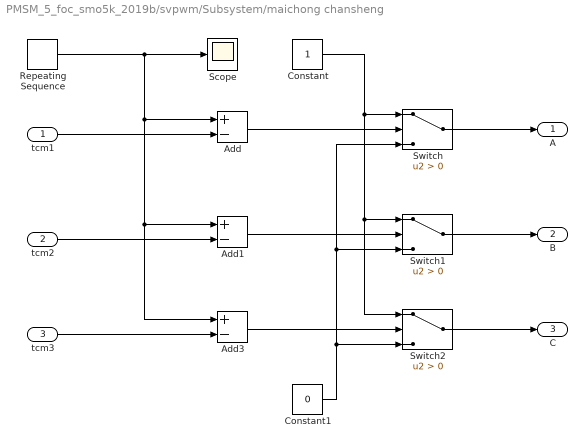
== system PMSM_5_foc_smo5k_2019b/svpwm/Subsystem/maichong chansheng ==
  tcm1 : Inport
  tcm2 : Inport  Port=2
  tcm3 : Inport  Port=3
  Add : Sum  Inputs=+-
  Add1 : Sum  Inputs=+-
  Add3 : Sum  Inputs=+-
  Constant : Constant
  Constant1 : Constant  Value=0
  Repeating Sequence : simulink/Sources/Repeating Sequence  rep_seq_t=[0 T/2 T]  rep_seq_y=[0 T/2 0]
  Scope : Scope
  Switch : Switch  Criteria=u2 > Threshold
  Switch1 : Switch  Criteria=u2 > Threshold
  Switch2 : Switch  Criteria=u2 > Threshold
  A : Outport
  B : Outport  Port=2
  C : Outport  Port=3
  wires:
  Repeating Sequence/1 -> Add1/1, Add3/1, Add/1, Scope/1
  tcm1/1 -> Add/2
  tcm2/1 -> Add1/2
  tcm3/1 -> Add3/2
  Constant/1 -> Switch2/1, Switch1/1, Switch/1
  Constant1/1 -> Switch/3, Switch1/3, Switch2/3
  Add/1 -> Switch/2
  Add1/1 -> Switch1/2
  Add3/1 -> Switch2/2
  Switch/1 -> A/1
  Switch1/1 -> B/1
  Switch2/1 -> C/1

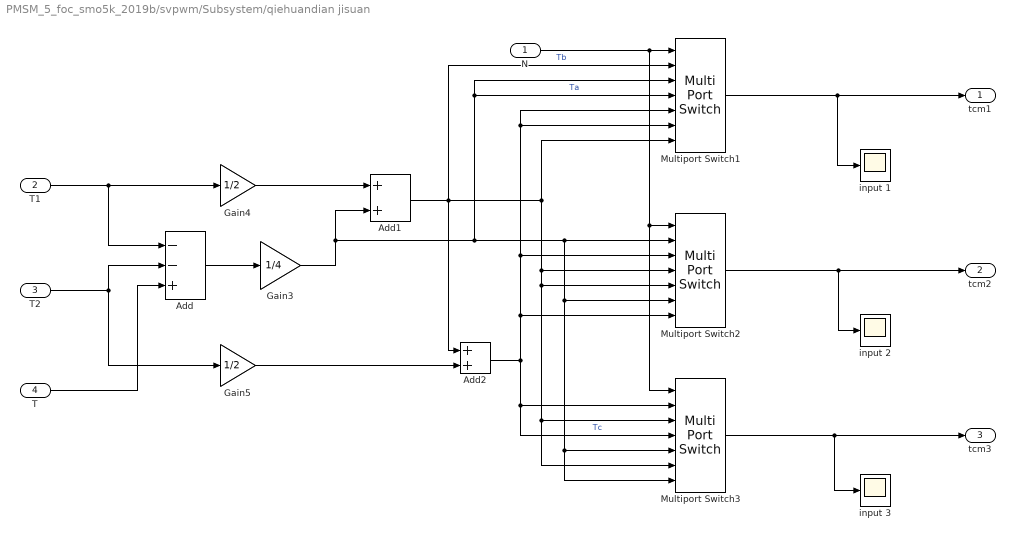
== system PMSM_5_foc_smo5k_2019b/svpwm/Subsystem/qiehuandian jisuan ==
  N : Inport
  T1 : Inport  Port=2
  T2 : Inport  Port=3
  T : Inport  Port=4
  Add : Sum  Inputs=--+
  Add1 : Sum
  Add2 : Sum
  Gain3 : Gain  Gain=1/4
  Gain4 : Gain  Gain=1/2
  Gain5 : Gain  Gain=1/2
  Multiport Switch1 : MultiPortSwitch  Inputs=6  DiagnosticForDefault=Warning
  Multiport Switch2 : MultiPortSwitch  Inputs=6  DiagnosticForDefault=Warning
  Multiport Switch3 : MultiPortSwitch  Inputs=6  DiagnosticForDefault=Warning
  input 1 : Scope
  input 2 : Scope
  input 3 : Scope
  tcm1 : Outport
  tcm2 : Outport  Port=2
  tcm3 : Outport  Port=3
  wires:
  T1/1 -> Add/1, Gain4/1
  T2/1 -> Gain5/1, Add/2
  T/1 -> Add/3
  Add/1 -> Gain3/1
  Gain3/1 -> Multiport Switch1/4, Multiport Switch1/3, Multiport Switch3/7, Multiport Switch3/5, Multiport Switch2/6, Multiport Switch2/2, Add1/2  "Ta"
  Gain4/1 -> Add1/1
  Add1/1 -> Add2/1, Multiport Switch2/4, Multiport Switch2/5, Multiport Switch3/3, Multiport Switch3/6, Multiport Switch1/7, Multiport Switch1/2  "Tb"
  Gain5/1 -> Add2/2
  Multiport Switch1/1 -> input 1/1, tcm1/1
  Multiport Switch3/1 -> input 3/1, tcm3/1
  N/1 -> Multiport Switch3/1, Multiport Switch2/1, Multiport Switch1/1
  Add2/1 -> Multiport Switch3/4, Multiport Switch3/2, Multiport Switch2/7, Multiport Switch1/6, Multiport Switch1/5, Multiport Switch2/3  "Tc"
  Multiport Switch2/1 -> input 2/1, tcm2/1

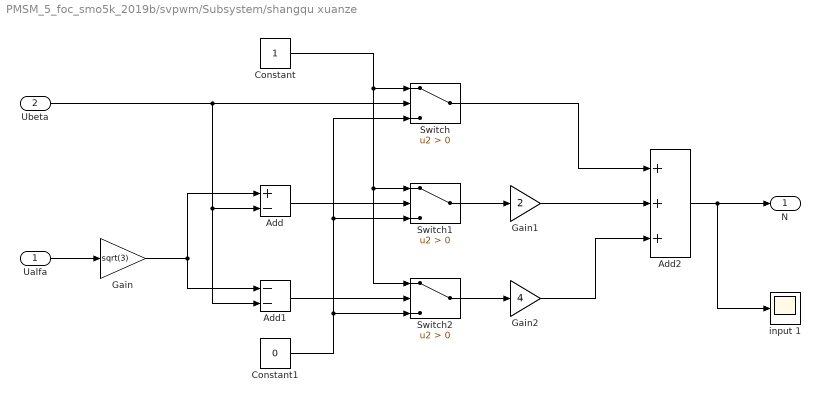
== system PMSM_5_foc_smo5k_2019b/svpwm/Subsystem/shangqu xuanze ==
  Ualfa : Inport
  Ubeta : Inport  Port=2
  Add : Sum  Inputs=+-
  Add1 : Sum  Inputs=--
  Add2 : Sum  Inputs=+++
  Constant : Constant
  Constant1 : Constant  Value=0
  Gain : Gain  Gain=sqrt(3)
  Gain1 : Gain  Gain=2
  Gain2 : Gain  Gain=4
  Switch : Switch  Criteria=u2 > Threshold
  Switch1 : Switch  Criteria=u2 > Threshold
  Switch2 : Switch  Criteria=u2 > Threshold
  input 1 : Scope
  N : Outport
  wires:
  Constant/1 -> Switch2/1, Switch1/1, Switch/1
  Ualfa/1 -> Gain/1
  Gain/1 -> Add1/1, Add/1
  Ubeta/1 -> Switch/2, Add1/2, Add/2
  Add/1 -> Switch1/2
  Constant1/1 -> Switch/3, Switch1/3, Switch2/3
  Add1/1 -> Switch2/2
  Switch1/1 -> Gain1/1
  Switch/1 -> Add2/1
  Gain1/1 -> Add2/2
  Gain2/1 -> Add2/3
  Add2/1 -> input 1/1, N/1
  Switch2/1 -> Gain2/1

== matlab function PMSM_5_foc_smo5k_2019b/MATLAB Function ==
  data: theta1 input; theta output
function theta = modtheta(theta1)
max=2*pi;min=-2*pi;
if(theta1>max)
    theta=(theta1/max-floor(theta1/max))*max;
elseif(theta1<min)
    theta=(theta1/min-floor(theta1/min))*min;
else
    theta=theta1;
end

== matlab function PMSM_5_foc_smo5k_2019b/filter2/ product ==
  data: kwr input; kk output; sat input
function kk = productkk(kwr,sat)

if(kwr>2)
    kk=1.5*kwr*sat;
else
    kk=10*sat;
end

== matlab function PMSM_5_foc_smo5k_2019b/filter2/ product1 ==
  data: kwr input; kk output; sat input
function kk = productkk(kwr,sat)

if(kwr>2)
    kk=1.5*kwr*sat;
else
    kk=10*sat;
end

== matlab function PMSM_5_foc_smo5k_2019b/filter2/complex filter/ccf ==
  data: we_input input; syalfa output; ealfa input; ebeta input; yalfa input; ybeta input; sybeta output; k_ccf input
function [syalfa,sybeta] = sat(we_input,ealfa,ebeta,yalfa,ybeta,k_ccf)
% we_input=abs(we_input);
if(we_input>10)
    syalfa=(ealfa-yalfa)*k_ccf*we_input-we_input*ebeta;
    sybeta=(ebeta-ybeta)*k_ccf*we_input+we_input*ealfa;
else
    syalfa=(ealfa-yalfa)*k_ccf*5-5*ebeta;
    sybeta=(ebeta-ybeta)*k_ccf*5+5*ealfa;
end

== matlab function PMSM_5_foc_smo5k_2019b/filter2/MATLAB Function2 ==
  data: theta1 input; theta output
function theta = modtheta(theta1)
max=2*pi;min=-2*pi;
% theta1=theta1+0;%atan(1/2);
if(theta1>max)
    theta1=(theta1/max-floor(theta1/max))*max;
elseif(theta1<min)
    theta1=(theta1/min-floor(theta1/min))*min;
end
theta=theta1;

== matlab function PMSM_5_foc_smo5k_2019b/MATLAB Function2 ==
  data: theta1 input; theta output
function theta = modtheta(theta1)
max=pi;min=-pi;
if(theta1>max)
    theta=theta1-2*max;
elseif(theta1<min)
    theta=theta1-2*min;
else
    theta=theta1;
end

== matlab function PMSM_5_foc_smo5k_2019b/MATLAB Function1 ==
  data: k input; TL output; wm input
function TL = TLGEN(k,wm)
    TL=k*wm^2;

== matlab function PMSM_5_foc_smo5k_2019b/pi /MATLAB Function1 ==
  data: postive_flag output; negative_flag output; y1 input; flag output; y2 input
function [postive_flag,negative_flag,flag] = panduan(y1,y2)
    if(y1>y2&&y1>0)
            postive_flag=1;
            negative_flag=0;
            flag=0;
            
    elseif(y1<y2&&y1<=0)
            postive_flag=0;
            negative_flag=1;
            flag=0;
    else
            postive_flag=0;
            negative_flag=0;
             flag=1;
    end

== matlab function PMSM_5_foc_smo5k_2019b/pi /MATLAB Function2 ==
  data: out output; postive_flag input; negative_flag input; flag input; error input
function out = panduan(postive_flag,negative_flag,flag,error)
    if(postive_flag==1&&error<0&&negative_flag==0&&flag==0)
        out=error;
    elseif(postive_flag==1&&error>=0&&negative_flag==0&&flag==0)
        out=0;
    elseif(negative_flag==1&&error<0&&postive_flag==0&&flag==0)
       out=0;
    elseif(negative_flag==1&&error>=0&&postive_flag==0&&flag==0)
        out=error;
    else
        out=error;
    end

== matlab function PMSM_5_foc_smo5k_2019b/pi 1/MATLAB Function1 ==
  data: postive_flag output; negative_flag output; y1 input; flag output; y2 input
function [postive_flag,negative_flag,flag] = panduan(y1,y2)
    if(y1>y2&&y1>0)
            postive_flag=1;
            negative_flag=0;
            flag=0;
            
    elseif(y1<y2&&y1<=0)
            postive_flag=0;
            negative_flag=1;
            flag=0;
    else
            postive_flag=0;
            negative_flag=0;
             flag=1;
    end

== matlab function PMSM_5_foc_smo5k_2019b/pi 1/MATLAB Function2 ==
  data: out output; postive_flag input; negative_flag input; flag input; error input
function out = panduan(postive_flag,negative_flag,flag,error)
    if(postive_flag==1&&error<0&&negative_flag==0&&flag==0)
        out=error;
    elseif(postive_flag==1&&error>=0&&negative_flag==0&&flag==0)
        out=0;
    elseif(negative_flag==1&&error<0&&postive_flag==0&&flag==0)
       out=0;
    elseif(negative_flag==1&&error>=0&&postive_flag==0&&flag==0)
        out=error;
    else
        out=error;
    end

== matlab function PMSM_5_foc_smo5k_2019b/pi 2/MATLAB Function1 ==
  data: postive_flag output; negative_flag output; y1 input; flag output; y2 input
function [postive_flag,negative_flag,flag] = panduan(y1,y2)
    if(y1>y2&&y1>0)
            postive_flag=1;
            negative_flag=0;
            flag=0;
            
    elseif(y1<y2&&y1<=0)
            postive_flag=0;
            negative_flag=1;
            flag=0;
    else
            postive_flag=0;
            negative_flag=0;
             flag=1;
    end

== matlab function PMSM_5_foc_smo5k_2019b/pi 2/MATLAB Function2 ==
  data: out output; postive_flag input; negative_flag input; flag input; error input
function out = panduan(postive_flag,negative_flag,flag,error)
    if(postive_flag==1&&error<0&&negative_flag==0&&flag==0)
        out=error;
    elseif(postive_flag==1&&error>=0&&negative_flag==0&&flag==0)
        out=0;
    elseif(negative_flag==1&&error<0&&postive_flag==0&&flag==0)
       out=0;
    elseif(negative_flag==1&&error>=0&&postive_flag==0&&flag==0)
        out=error;
    else
        out=error;
    end
